simulink library "INT_TCPrt_TrqLim"  (R2016b)
settings: Solver=VariableStepAuto  StartTime=0.0  StopTime=10.0  RelTol=1e-3
settings Model: Creator=Administrator  LastModifiedBy=Administrator

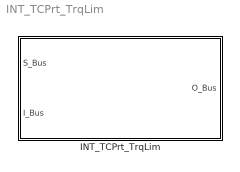
== system INT_TCPrt_TrqLim ==
  INT_TCPrt_TrqLim : Subsystem

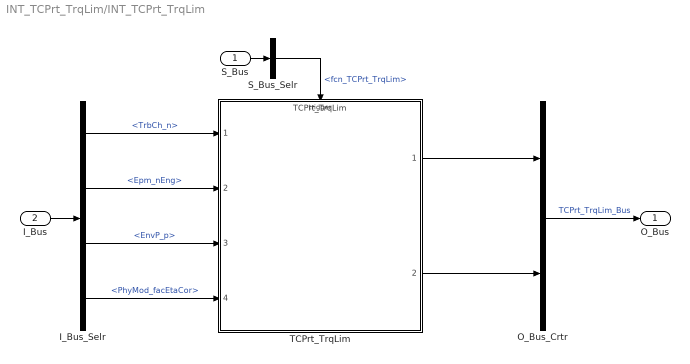
== system INT_TCPrt_TrqLim/INT_TCPrt_TrqLim ==
  S_Bus : Inport
  I_Bus : Inport  Port=2
  I_Bus_Selr : BusSelector  OutputSignals=TrbCh_n,Epm_nEng,EnvP_p,PhyMod_facEtaCor
  O_Bus_Crtr : BusCreator  Inputs=2
  S_Bus_Selr : BusSelector  OutputSignals=fcn_TCPrt_TrqLim
  TCPrt_TrqLim : ModelReference  ModelNameDialog=TCPrt_TrqLim  SimulationMode=Normal  ModelReferenceVersion=1.14  TriggerPortName=function  TriggerPortTriggerType=function-call  TriggerPortStatesWhenEnabling=held
  O_Bus : Outport
  wires:
  S_Bus_Selr/1 -> TCPrt_TrqLim/Trigger  "<fcn_TCPrt_TrqLim>"
  S_Bus/1 -> S_Bus_Selr/1
  I_Bus/1 -> I_Bus_Selr/1
  I_Bus_Selr/1 -> TCPrt_TrqLim/1  "<TrbCh_n>"
  I_Bus_Selr/2 -> TCPrt_TrqLim/2  "<Epm_nEng>"
  I_Bus_Selr/3 -> TCPrt_TrqLim/3  "<EnvP_p>"
  I_Bus_Selr/4 -> TCPrt_TrqLim/4  "<PhyMod_facEtaCor>"
  O_Bus_Crtr/1 -> O_Bus/1  "TCPrt_TrqLim_Bus"
  TCPrt_TrqLim/1 -> O_Bus_Crtr/1
  TCPrt_TrqLim/2 -> O_Bus_Crtr/2
